simulink model "CompareToConstant_TestGen21"  (R2017b)
settings: Solver=FixedStepDiscrete  StartTime=0.0  StopTime=10.0  RelTol=1e-3
undefined symbols (not defined in the file): Block_TestLib, enable
libraries: simulink x1
settings Model: Creator=ktrinh  LastModifiedBy=ktrinh
settings DebuggingCC: ParameterOverflowMsg=none

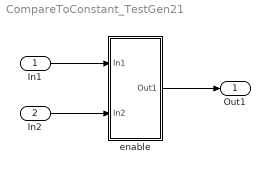
== system CompareToConstant_TestGen21 ==
  In1 : Inport
  In2 : Inport  Port=2
  enable : Subsystem  AncestorBlock=Block_TestLib/enable
  Out1 : Outport
  wires:
  In1/1 -> enable/1(In1)
  In2/1 -> enable/2(In2)
  enable/1(Out1) -> Out1/1

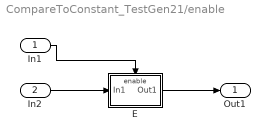
== system CompareToConstant_TestGen21/enable ==
  In1 : Inport  OutDataTypeStr=boolean
  In2 : Inport  Port=2
  E : Subsystem  TreatAsAtomicUnit=on
  Out1 : Outport
  wires:
  In1/1 -> E/Enable
  In2/1 -> E/1(In1)
  E/1(Out1) -> Out1/1

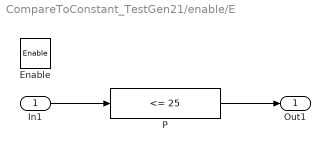
== system CompareToConstant_TestGen21/enable/E ==
  In1 : Inport  OutDataTypeStr=int8  PortDimensions=1
  Enable : EnablePort
  P : simulink/Logic and Bit Operations/Compare To Constant  relop=<=  const=25  OutDataTypeStr=uint8
  Out1 : Outport
  wires:
  In1/1 -> P/1
  P/1 -> Out1/1
